simulink model "BLDC_dq_Control_abcModel"  (R2021a)
settings: Solver=FixedStepAuto  StartTime=0.0  StopTime=10  FixedStep=0.00001  RelTol=1e-3
undefined symbols (not defined in the file): sigbuilder_block
libraries: pid_lib x3
settings Model: Creator=raca  LastModifiedBy=headl
settings SolverCC: AlgebraicLoopSolver=TrustRegion
settings DataIOCC: ReturnWorkspaceOutputs=off
settings DebuggingCC: SFMachineParentedDataDiag=warning  ArithmeticOperatorsInVariantConditions=warning
settings SFSimCC: SimUseLocalCustomCode=off  CustomCodeUndefinedFunction=UseInterfaceOnly
settings RTWCC: RTWUseLocalCustomCode=off
settings CodeAppCC: StateflowObjectComments=on

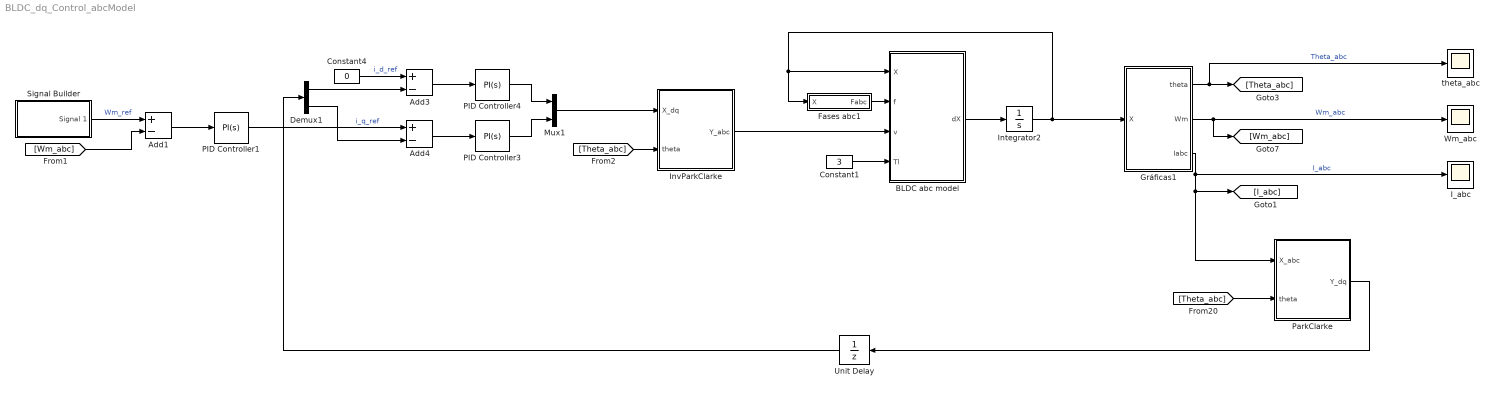
== system BLDC_dq_Control_abcModel ==
  Add1 : Sum  Inputs=+-
  Add3 : Sum  Inputs=+-
  Add4 : Sum  Inputs=+-
  BLDC abc model : MATLAB Function  TreatAsAtomicUnit=on
  Constant1 : Constant  Value=3
  Constant4 : Constant  Value=0
  Demux1 : Demux  Outputs=2
  Fases abc1 : MATLAB Function  TreatAsAtomicUnit=on
  Gráficas1 : MATLAB Function  TreatAsAtomicUnit=on
  I_abc : Scope
  Integrator2 : Integrator  InitialCondition=[0;0;0;1;0]
  InvParkClarke : MATLAB Function  TreatAsAtomicUnit=on
  Mux1 : Mux  Inputs=2
  PID Controller1 : pid_lib/PID Controller  Controller=PI  Form=Parallel  TimeDomain=Continuous-time  UseExternalTs=off  SampleTime=-1  IntegratorMethod=Forward Euler  FilterMethod=Forward Euler  ControllerParametersSource=internal  P=-0.310960961217836  I=-13.7967942361801  D=0  UseFilter=on  N=100  TunerSelectOption=Transfer Function Based (PID Tuner App)  InitialConditionSource=internal  InitialConditionForIntegrator=0  InitialConditionForFilter=0  DifferentiatorICPrevScaledInput=0  ExternalReset=none  TrackingMode=off  Kt=1  LimitOutput=off  SatLimitsSource=internal  UpperSaturationLimit=inf  LowerSaturationLimit=-inf  LinearizeAsGain=on  AntiWindupMode=none  Kb=1  POutMin=[]  POutMax=[]  IOutMin=[]  IOutMax=[]  DOutMin=[]  DOutMax=[]  NOutMin=[]  NOutMax=[]  SumOutMin=[]  SumOutMax=[]  SaturationOutMin=[]  SaturationOutMax=[]  PParamMin=[]  PParamMax=[]  IParamMin=[]  IParamMax=[]  DParamMin=[]  DParamMax=[]  NParamMin=[]  NParamMax=[]  KbParamMin=[]  KbParamMax=[]  KtParamMin=[]  KtParamMax=[]  KbOutMin=[]  KbOutMax=[]  KtOutMin=[]  KtOutMax=[]  IntegratorOutMin=[]  IntegratorOutMax=[]  FilterOutMin=[]  FilterOutMax=[]  SumI1OutMin=[]  SumI1OutMax=[]  SumI2OutMin=[]  SumI2OutMax=[]  SumI3OutMin=[]  SumI3OutMax=[]  SumI4OutMin=[]  SumI4OutMax=[]  SumDOutMin=[]  SumDOutMax=[]  DifferentiatorOutMin=[]  DifferentiatorOutMax=[]  FilterDiffOutCoefMin=[]  FilterDiffOutCoefMax=[]  ReciprocalOutMin=[]  ReciprocalOutMax=[]  SumDenOutMin=[]  SumDenOutMax=[]  SumNumOutMin=[]  SumNumOutMax=[]  DivideOutMin=[]  DivideOutMax=[]  UdiffTsProdOutMin=[]  UdiffTsProdOutMax=[]  NTsProdOutMin=[]  NTsProdOutMax=[]  UintegralTsProdOutMin=[]  UintegralTsProdOutMax=[]  UngainTsProdOutMin=[]  UngainTsProdOutMax=[]  IntegratorContinuousStateAttributes=''  IntegratorStateMustResolveToSignalObject=off  IntegratorRTWStateStorageClass=Auto  FilterContinuousStateAttributes=''  FilterStateMustResolveToSignalObject=off  FilterRTWStateStorageClass=Auto  ParallelPVariant=InternalParameters  IdealPVariant=Disabled  IVariant=InternalParameters  DVariant=Disabled  IntegratorVariant=Continuous  SatVariant=Disabled  AWVariant=Passthrough  PCopyVariant=Disabled  TRVariant=Disabled  FdbkBlocksVariant=Forward  IdealPFdbkVariant=Disabled  SatFdbkVariant=Disabled  DerivativeFilterVariant=Disabled  NVariant=Disabled  NCopyVariant=Disabled_SignalSpec  FilterICVariant=Disabled  IntegratorICVariant=InternalICs  ExternalResetVariant=Disabled  TRSumVariant=Passthrough  SumFdbkVariant=Disabled  SumVariant=Sum_PI  TsampFilterVariant=InternalTs  TsampNgainVariant=Passthrough  TsampIntegralVariant=Passthrough  ExternalSaturationOutDataTypeStr=Inherit: Same as second input
  PID Controller3 : pid_lib/PID Controller  Controller=PI  Form=Parallel  TimeDomain=Continuous-time  UseExternalTs=off  SampleTime=-1  IntegratorMethod=Forward Euler  FilterMethod=Forward Euler  ControllerParametersSource=internal  P=0  I=123.656555611116  D=0  UseFilter=on  N=100  TunerSelectOption=Transfer Function Based (PID Tuner App)  InitialConditionSource=internal  InitialConditionForIntegrator=0  InitialConditionForFilter=0  DifferentiatorICPrevScaledInput=0  ExternalReset=none  TrackingMode=off  Kt=1  LimitOutput=off  SatLimitsSource=internal  UpperSaturationLimit=inf  LowerSaturationLimit=-inf  LinearizeAsGain=on  AntiWindupMode=none  Kb=1  POutMin=[]  POutMax=[]  IOutMin=[]  IOutMax=[]  DOutMin=[]  DOutMax=[]  NOutMin=[]  NOutMax=[]  SumOutMin=[]  SumOutMax=[]  SaturationOutMin=[]  SaturationOutMax=[]  PParamMin=[]  PParamMax=[]  IParamMin=[]  IParamMax=[]  DParamMin=[]  DParamMax=[]  NParamMin=[]  NParamMax=[]  KbParamMin=[]  KbParamMax=[]  KtParamMin=[]  KtParamMax=[]  KbOutMin=[]  KbOutMax=[]  KtOutMin=[]  KtOutMax=[]  IntegratorOutMin=[]  IntegratorOutMax=[]  FilterOutMin=[]  FilterOutMax=[]  SumI1OutMin=[]  SumI1OutMax=[]  SumI2OutMin=[]  SumI2OutMax=[]  SumI3OutMin=[]  SumI3OutMax=[]  SumI4OutMin=[]  SumI4OutMax=[]  SumDOutMin=[]  SumDOutMax=[]  DifferentiatorOutMin=[]  DifferentiatorOutMax=[]  FilterDiffOutCoefMin=[]  FilterDiffOutCoefMax=[]  ReciprocalOutMin=[]  ReciprocalOutMax=[]  SumDenOutMin=[]  SumDenOutMax=[]  SumNumOutMin=[]  SumNumOutMax=[]  DivideOutMin=[]  DivideOutMax=[]  UdiffTsProdOutMin=[]  UdiffTsProdOutMax=[]  NTsProdOutMin=[]  NTsProdOutMax=[]  UintegralTsProdOutMin=[]  UintegralTsProdOutMax=[]  UngainTsProdOutMin=[]  UngainTsProdOutMax=[]  IntegratorContinuousStateAttributes=''  IntegratorStateMustResolveToSignalObject=off  IntegratorRTWStateStorageClass=Auto  FilterContinuousStateAttributes=''  FilterStateMustResolveToSignalObject=off  FilterRTWStateStorageClass=Auto  ParallelPVariant=InternalParameters  IdealPVariant=Disabled  IVariant=InternalParameters  DVariant=Disabled  IntegratorVariant=Continuous  SatVariant=Disabled  AWVariant=Passthrough  PCopyVariant=Disabled  TRVariant=Disabled  FdbkBlocksVariant=Forward  IdealPFdbkVariant=Disabled  SatFdbkVariant=Disabled  DerivativeFilterVariant=Disabled  NVariant=Disabled  NCopyVariant=Disabled_SignalSpec  FilterICVariant=Disabled  IntegratorICVariant=InternalICs  ExternalResetVariant=Disabled  TRSumVariant=Passthrough  SumFdbkVariant=Disabled  SumVariant=Sum_PI  TsampFilterVariant=InternalTs  TsampNgainVariant=Passthrough  TsampIntegralVariant=Passthrough  ExternalSaturationOutDataTypeStr=Inherit: Same as second input
  PID Controller4 : pid_lib/PID Controller  Controller=PI  Form=Parallel  TimeDomain=Continuous-time  UseExternalTs=off  SampleTime=-1  IntegratorMethod=Forward Euler  FilterMethod=Forward Euler  ControllerParametersSource=internal  P=0.854442807084617  I=1483.79827419022  D=0  UseFilter=on  N=100  TunerSelectOption=Transfer Function Based (PID Tuner App)  InitialConditionSource=internal  InitialConditionForIntegrator=0  InitialConditionForFilter=0  DifferentiatorICPrevScaledInput=0  ExternalReset=none  TrackingMode=off  Kt=1  LimitOutput=off  SatLimitsSource=internal  UpperSaturationLimit=inf  LowerSaturationLimit=-inf  LinearizeAsGain=on  AntiWindupMode=none  Kb=1  POutMin=[]  POutMax=[]  IOutMin=[]  IOutMax=[]  DOutMin=[]  DOutMax=[]  NOutMin=[]  NOutMax=[]  SumOutMin=[]  SumOutMax=[]  SaturationOutMin=[]  SaturationOutMax=[]  PParamMin=[]  PParamMax=[]  IParamMin=[]  IParamMax=[]  DParamMin=[]  DParamMax=[]  NParamMin=[]  NParamMax=[]  KbParamMin=[]  KbParamMax=[]  KtParamMin=[]  KtParamMax=[]  KbOutMin=[]  KbOutMax=[]  KtOutMin=[]  KtOutMax=[]  IntegratorOutMin=[]  IntegratorOutMax=[]  FilterOutMin=[]  FilterOutMax=[]  SumI1OutMin=[]  SumI1OutMax=[]  SumI2OutMin=[]  SumI2OutMax=[]  SumI3OutMin=[]  SumI3OutMax=[]  SumI4OutMin=[]  SumI4OutMax=[]  SumDOutMin=[]  SumDOutMax=[]  DifferentiatorOutMin=[]  DifferentiatorOutMax=[]  FilterDiffOutCoefMin=[]  FilterDiffOutCoefMax=[]  ReciprocalOutMin=[]  ReciprocalOutMax=[]  SumDenOutMin=[]  SumDenOutMax=[]  SumNumOutMin=[]  SumNumOutMax=[]  DivideOutMin=[]  DivideOutMax=[]  UdiffTsProdOutMin=[]  UdiffTsProdOutMax=[]  NTsProdOutMin=[]  NTsProdOutMax=[]  UintegralTsProdOutMin=[]  UintegralTsProdOutMax=[]  UngainTsProdOutMin=[]  UngainTsProdOutMax=[]  IntegratorContinuousStateAttributes=''  IntegratorStateMustResolveToSignalObject=off  IntegratorRTWStateStorageClass=Auto  FilterContinuousStateAttributes=''  FilterStateMustResolveToSignalObject=off  FilterRTWStateStorageClass=Auto  ParallelPVariant=InternalParameters  IdealPVariant=Disabled  IVariant=InternalParameters  DVariant=Disabled  IntegratorVariant=Continuous  SatVariant=Disabled  AWVariant=Passthrough  PCopyVariant=Disabled  TRVariant=Disabled  FdbkBlocksVariant=Forward  IdealPFdbkVariant=Disabled  SatFdbkVariant=Disabled  DerivativeFilterVariant=Disabled  NVariant=Disabled  NCopyVariant=Disabled_SignalSpec  FilterICVariant=Disabled  IntegratorICVariant=InternalICs  ExternalResetVariant=Disabled  TRSumVariant=Passthrough  SumFdbkVariant=Disabled  SumVariant=Sum_PI  TsampFilterVariant=InternalTs  TsampNgainVariant=Passthrough  TsampIntegralVariant=Passthrough  ExternalSaturationOutDataTypeStr=Inherit: Same as second input
  ParkClarke : MATLAB Function  TreatAsAtomicUnit=on
  Signal Builder : Subsystem  Tag=STV Subsys  LoadFcn=sigbuilder_block('load');  StartFcn=sigbuilder_block('start');  StopFcn=sigbuilder_block('stop');  ClipboardFcn=sigbuilder_block('clipboard');  mask(Sigbuilder block){tuvar=[0:10]}
      mask help: Simulink:masks:SigbuilderBlock_MD
      mask init:
      | if ~strcmp(get_param(bdroot(gcbh),'SimulationStatus'),'stopped') tuvar = sigbuilder_block('maskInit'); end
      settings: CopyFcn=sigbuilder_block('copy');  DeleteFcn=sigbuilder_block('delete');  ModelCloseFcn=sigbuilder_block('modelClose');  PreSaveFcn=sigbuilder_block('preSave');  PauseFcn=sigbuilder_block('pause');  ContinueFcn=sigbuilder_block('continue');  NameChangeFcn=sigbuilder_block('namechange');  OpenFcn=sigbuilder_block('open',[437.6 199.2 550.4 400 ]);  CloseFcn=sigbuilder_block('close');
      mask Display: plot(0, 0, 100, 100,[2, 2, 32, 32, 2], [68, 8, 8, 68, 68],[32, 2], [38, 38], [32, 19, 2],[53, 60, 44], [32, 17, 17, 2],[16, 16, 31, 31]);txt = getActiveGroup(gcbh);text(2, 100, txt,'verticalAlignment', 'top');
  Unit Delay : UnitDelay  SampleTime=-1  HasFrameUpgradeWarning=on
  Wm_abc : Scope
  theta_abc : Scope
  wires:
  Constant4/1 -> Add3/1  "i_d_ref"
  Add4/1 -> PID Controller3/1
  Add3/1 -> PID Controller4/1
  Demux1/2 -> Add4/2
  Demux1/1 -> Add3/2
  PID Controller4/1 -> Mux1/1
  PID Controller3/1 -> Mux1/2
  Unit Delay/1 -> Demux1/1
  Add1/1 -> PID Controller1/1
  [Wm_abc] -> Add1/2
  PID Controller1/1 -> Add4/1  "i_q_ref"
  Signal Builder/1(Signal 1) -> Add1/1  "Wm_ref"
  Gráficas1/2(Wm) -> [Wm_abc], Wm_abc/1  "Wm_abc"
  Integrator2/1 -> Gráficas1/1(X), BLDC abc model/1(X), Fases abc1/1(X)
  Fases abc1/1(Fabc) -> BLDC abc model/2(f)
  Constant1/1 -> BLDC abc model/4(Tl)
  Gráficas1/1(theta) -> theta_abc/1, [Theta_abc]  "Theta_abc"
  BLDC abc model/1(dX) -> Integrator2/1
  Gráficas1/3(Iabc) -> [I_abc], ParkClarke/1(X_abc), I_abc/1  "I_abc"
  Mux1/1 -> InvParkClarke/1(X_dq)
  InvParkClarke/1(Y_abc) -> BLDC abc model/3(v)
  [Theta_abc] -> InvParkClarke/2(theta)
  [Theta_abc] -> ParkClarke/2(theta)
  ParkClarke/1(Y_dq) -> Unit Delay/1

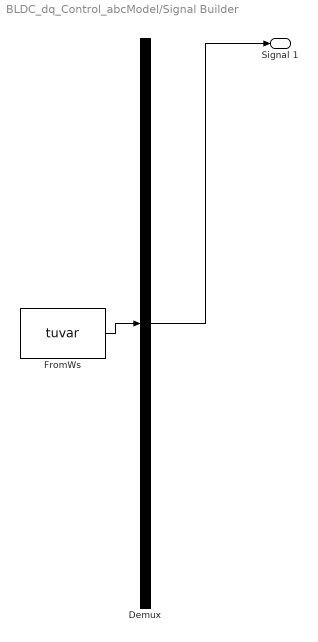
== system BLDC_dq_Control_abcModel/Signal Builder ==
  Demux : Demux  Tag=STV Demux  Outputs=1
      settings: DisplayOption=none
  FromWs : FromWorkspace  Tag=STV FromWs  VariableName=tuvar
      SigBuilderData=|
      | common.afterFinalStr = 'Extrapolate'
      | common.sampleTime = 0
      | dataSet.timeRange = [0 10]
      | dataSet.name = 'Group 1'
      | sbobj.Groups.Name = 'Group 1'
      | sbobj.Groups.Signals.Name = 'Signal 1'
      | sbobj.Groups.Signals.XData = [0 4 4 6 10]
      | sbobj.Groups.Signals.YData = [4 4 15 15 4]
  Signal 1 : Outport  Tag=STV Outport
  wires:
  Demux/1 -> Signal 1/1
  FromWs/1 -> Demux/1

== matlab function BLDC_dq_Control_abcModel/Fases abc1 ==
  data: X input; Fabc output
function Fabc = fcn(X)
Fabc = [0;0;0];
    theta = mod(X(5),2*pi); %X(4)
    %theta = mod(X,2*pi);
    
    if (0<=theta)&&(theta<(pi/6))
        Fa = (6/pi)*theta;
    elseif ((pi/6)<=theta)&&(theta<(5*pi/6))
        Fa = 1;
    elseif ((5*pi/6<=theta))&&(theta<(7*pi/6))
        Fa = (6/pi)*(pi-theta);
    elseif ((7*pi/6)<=theta)&&(theta<(11*pi/6))
        Fa = -1;
    elseif ((11*pi/6)<=theta)&&(theta<(2*pi))
        Fa = (6/pi)*(theta-2*pi);
    else
        Fa = NaN;
    end
    
    if (0<=theta)&&(theta<(3*pi/6))
        Fb = -1;
    elseif ((3*pi/6)<=theta)&&(theta<(5*pi/6))
        Fb = (6/pi)*(theta-(2*pi)/3);
    elseif ((5*pi/6)<=theta)&&(theta<(9*pi/6))
        Fb = 1;
    elseif ((9*pi/6)<=theta)&&(theta<(11*pi/6))
        Fb = (6/pi)*(-theta+(5*pi)/3);
    elseif ((11*pi/6)<=theta)&&(theta<(2*pi))
        Fb = -1;
    else
        Fb = NaN;
    end
    
    if (0<=theta)&&(theta<(pi/6))
        Fc = 1;
    elseif ((pi/6)<=theta)&&(theta<(3*pi/6))
        Fc = (6/pi)*(pi/3-theta);
    elseif ((3*pi/6)<=theta)&&(theta<(7*pi/6))
        Fc = -1;
    elseif ((7*pi/6)<=theta)&&(theta<(9*pi/6))
        Fc = (6/pi)*(theta-(4*pi)/3);
    elseif ((9*pi/6)<=theta)&&(theta<(2*pi))
        Fc = 1;
    else
        Fc = NaN; 
    end
    
    
%     
     Fa = sin(theta);
     Fb = sin(theta - 2*pi/3);
     Fc = sin(theta + 2*pi/3);
    
    Fabc = [Fa;Fb;Fc];
end

== matlab function BLDC_dq_Control_abcModel/BLDC abc model ==
  data: X input; f input; v input; dX output; Tl input
function dX = fcn(X,f,v,Tl)
u = [v;Tl]; 
i_a = X(1); i_b = X(2); i_c = X(3); wm = X(4); theta = X(5);

lambda = 0.0433;
R = 0.35;
L = 0.001;
M = 0.000;
J = 0.00018;
P = 4;
b = 0.0034;

%e = [(lamda*wm).*f;0;0];

A =[-(R/(L-M)) 0 0 -(lambda/(L-M))*f(1) 0;...
    0 -(R/(L-M)) 0 -(lambda/(L-M))*f(2) 0;...
    0 0 -(R/(L-M)) -(lambda/(L-M))*f(3) 0;...
    (lambda/J)*f(1) (lambda/J)*f(2) (lambda/J)*f(3) -b/J 0;...
    0 0 0 P/2 0];

B = diag([1/(L-M) 1/(L-M) 1/(L-M) -1/J]);
B = [B;0 0 0 0];


dX = [0;0;0;0;0];
dX = A*X + B*u;

end

== matlab function BLDC_dq_Control_abcModel/Gráficas1 ==
  data: X input; theta output; Wm output; Iabc output
function [theta,Wm,Iabc] = DEMUX(X)
theta = X(5); Wm = X(4);Iabc = X(1:3);

== matlab function BLDC_dq_Control_abcModel/InvParkClarke ==
  data: X_dq input; Y_abc output; theta input
function Y_abc = fcn(X_dq, theta)
X_dq0 = [X_dq;0];

%inverse Park-Clarke power invariant
iT_PC = sqrt(2/3)*[cos(theta)          -sin(theta)            1/sqrt(2); ...
                  cos(theta-2*pi/3)   -sin(theta-2*pi/3)     1/sqrt(2); ...
                  cos(theta+2*pi/3)   -sin(theta+2*pi/3)     1/sqrt(2)];
%               
              
 %inverse Park-Clarke amplitude invariant
% iT_PC = [cos(theta)          -sin(theta)            1; ...
%          cos(theta-2*pi/3)   -sin(theta-2*pi/3)     1; ...
%          cos(theta+2*pi/3)   -sin(theta+2*pi/3)     1];



Y_abc =iT_PC*X_dq0;
end

== matlab function BLDC_dq_Control_abcModel/ParkClarke ==
  data: X_abc input; Y_dq output; theta input
function Y_dq = fcn(X_abc, theta)

% Park clarke transform eliminating the third element
PC_T = (sqrt(2)/2)*[sqrt(3)*cos(theta)  sin(theta)  -sin(theta) ; ...
                    -sqrt(3)*sin(theta)  cos(theta)  -cos(theta)];

Y_dq =PC_T*X_abc;
end
